simulink model "quad_integrator_subsys"  (Simulink 7.3)
settings: Solver=ode45  StartTime=0.0  StopTime=10*30  FixedStep=.0001  MaxStep=.02  RelTol=1e-3
InitFcn:
  | Ts=0.02;
settings Model: Creator=jporter  LastModifiedBy=jporter
settings OptimizationCC: InitFltsAndDblsToZero=on

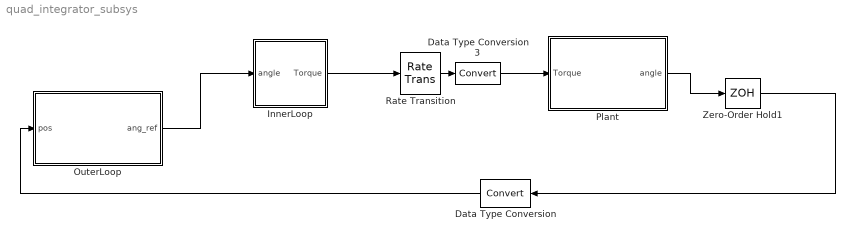
== system quad_integrator_subsys ==
  Data Type Conversion : DataTypeConversion  OutDataType=sfix(16)  OutScaling=2^0
  Data Type Conversion3 : DataTypeConversion  OutDataType=sfix(16)  OutScaling=2^0
  InnerLoop : Subsystem
  OuterLoop : Subsystem
  Plant : Subsystem
  Rate Transition : RateTransition
  Zero-Order Hold1 : ZeroOrderHold  SampleTime=Ts
  wires:
  InnerLoop/1(Torque) -> Rate Transition/1
  Data Type Conversion/1 -> OuterLoop/1(pos)
  Data Type Conversion3/1 -> Plant/1(Torque)
  Rate Transition/1 -> Data Type Conversion3/1
  Zero-Order Hold1/1 -> Data Type Conversion/1
  Plant/1(angle) -> Zero-Order Hold1/1
  OuterLoop/1(ang_ref) -> InnerLoop/1(angle)

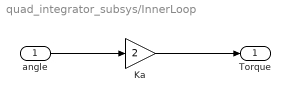
== system quad_integrator_subsys/InnerLoop ==
  angle : Inport  DataType=single  OutDataTypeStr=single
  Ka : Gain  Gain=2  ParameterDataTypeMode=single  ParameterDataType=sfix(16)  ParameterScaling=2^0  ParamDataTypeStr=single  OutDataType=sfix(16)  OutScaling=2^0
  Torque : Outport  DataType=single  OutDataTypeStr=single
  wires:
  angle/1 -> Ka/1
  Ka/1 -> Torque/1

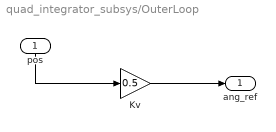
== system quad_integrator_subsys/OuterLoop ==
  pos : Inport  DataType=single  OutDataTypeStr=single
  Kv : Gain  Gain=0.5  ParameterDataTypeMode=single  ParameterDataType=sfix(16)  ParameterScaling=2^0  ParamDataTypeStr=single  OutDataType=sfix(16)  OutScaling=2^0
  ang_ref : Outport  DataType=single  OutDataTypeStr=single
  wires:
  Kv/1 -> ang_ref/1
  pos/1 -> Kv/1

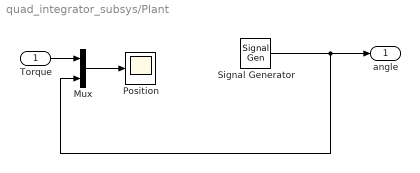
== system quad_integrator_subsys/Plant ==
  Torque : Inport
  Mux : Mux  Inputs=2
  Position : Scope
      settings: YMin=-20  YMax=20  SaveName=ScopeData7
  Signal Generator : SignalGenerator  Frequency=1/30
  angle : Outport
  wires:
  Signal Generator/1 -> angle/1, Mux/2
  Torque/1 -> Mux/1
  Mux/1 -> Position/1
